simulink model "scalarsdesmc"  (R2020a)
settings: Solver=FixedStepAuto  StartTime=0.0  StopTime=10.0  FixedStep=1e-2  MaxStep=1e-1  RelTol=1e-12  EnableMultiTasking=on
settings Model: Creator=amal029_old  LastModifiedBy=amal029_old
settings SolverCC: ZeroCrossAlgorithm=Adaptive  AutoInsertRateTranBlk=on
settings DataIOCC: LimitDataPoints=on  ReturnWorkspaceOutputs=off
settings OptimizationCC: LifeSpan=inf
settings DebuggingCC: AllowSymbolicDim=off  SFUnexpectedBacktrackingDiag=warning  SFNoUnconditionalDefaultTransitionDiag=warning  SFExecutionAtInitializationDiag=none  ArithmeticOperatorsInVariantConditions=warning
settings SFSimCC: SimUseLocalCustomCode=off  CustomCodeUndefinedFunction=UseInterfaceOnly
settings RTWCC: RTWUseLocalCustomCode=off
settings CodeAppCC: StateflowObjectComments=on
settings GRTTargetCC: TargetLangStandard=C89/C90 (ANSI)
settings ConfigComp: CovMetricSettings=dw  CovHtmlReporting=on  CovSaveCumulativeToWorkspaceVar=on  CovSaveSingleToWorkspaceVar=on  CovShowResultsExplorer=off  CovExternalEMLEnable=off

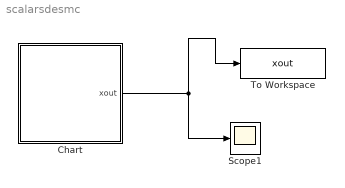
== system scalarsdesmc ==
  Chart : Stateflow chart  TreatAsAtomicUnit=on
  Scope1 : Scope
  To Workspace : ToWorkspace  VariableName=xout  SaveFormat=Structure With Time  SampleTime=-1
  wires:
  Chart/1(xout) -> To Workspace/1, Scope1/1

== stateflow chart scalarsdesmc/Chart ==
  settings: description=This is example of a very simple sliding mode controller
  state State2
    du:
    x=x+0.01*D-normrnd(0, sqrt(D));
    xout=x;
  state State3
    du:
    xout=x;
  state State1
    du:
    x=x-0.01*D+normrnd(0, sqrt(D));
    xout = x;
  (default) -> State2 [order 1] : [x<pi/2]{ xout=x; rng('shuffle')}
  State2 -> State3 [order 1] : [cos(x) >= 0 && cos(x) <= epsilon]
  State1 -> State2 [order 2] : [cos(x) >= epsilon]
  State2 -> State1 [order 2] : [cos(x)  <= -epsilon]
  (default) -> State1 [order 2] : {xout=x; rng('shuffle')}
  State1 -> State3 [order 1] : [cos(x) >= -epsilon && cos(x) <= 0 ]
  data: x local =0.5; xout output; epsilon constant double =1e-1; D constant double =1e-2
  data x settings: updateMethod=SF_CONTINUOUS_TIME_DATA
